simulink model "modeloKevin"  (R2017b)
settings: Solver=VariableStepAuto  StartTime=0.0  StopTime=200  RelTol=1e-3
values from neighbouring files (symbols this model uses):
  Awr = 0.0058    [variablesms.m]
  b = 0.0000000001    (= 1e-10)    [variablesms.m]
  Bi = 0.1    [variablesms.m]
  c = 0.012    [variablesms.m]
  CargaR = 1000    [variablesms.m]
  cpg = 1006    [variablesms.m]
  cpv = 1873.3    [variablesms.m]
  cpw = 4227    [variablesms.m]
  dg = 1.23    [variablesms.m]
  dv = 14.71    [variablesms.m]
  dw = 1000    [variablesms.m]
  F1 = 0.001    [variablesms.m]
  F2 = 0.001    [variablesms.m]
  fve = 60/(2*pi())    [variablesms.m]
  h = 1000    [variablesms.m]
  J = 0.004    [variablesms.m]
  Ji = 1.72    [variablesms.m]
  Kb = 6.2    [variablesms.m]
  Kp = 5.6627    [variablesms.m]
  l = 0.06    [variablesms.m]
  L_d = 38e-3    (= 0.038)    [variablesms.m]
  L_q = 9.03e-3    (= 0.00903)    [variablesms.m]
  Lambda = 0.48    [variablesms.m]
  P = 1    [variablesms.m]
  Patm = 101.325    [variablesms.m]
  r = 0.02    [variablesms.m]
  Rg = 0.287    [variablesms.m]
  Ri = 0.973    [variablesms.m]
  rp = 0.015    [variablesms.m]
  Rs = 1.649    [variablesms.m]
  Tcold = 300    [variablesms.m]
  Thot = 600    [variablesms.m]
  V1 = 0.001    [variablesms.m]
  V2 = 0.001    [variablesms.m]
undefined symbols (not defined in the file or in its folder): sigbuilder_block
libraries: powerlib_meascontrol x1, simulink x1
settings Model: Creator=Osorio  LastModifiedBy=Hp 14
settings CodeAppCC: StateflowObjectComments=on

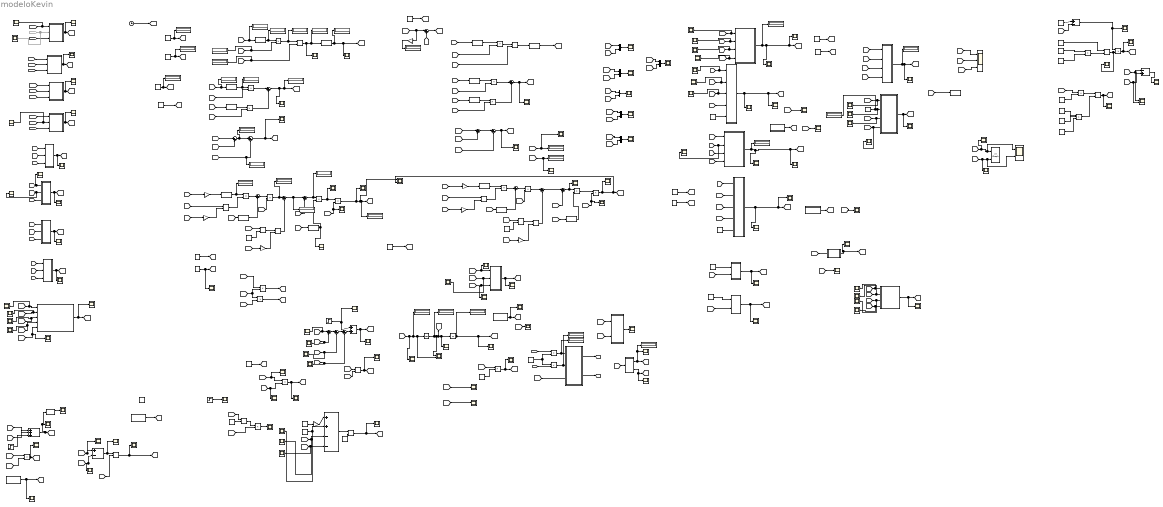
== system modeloKevin ==
  note: RORE AMARILLO
      | TORC AZUL
  note: ECUACION 30
  note: ECUACION 29
  note: ECUACION 27
  note: ECUACION 28
  note: ECUACION 24
  note: ECUACIO 25
  note: ECUACION 22
  note: ECUACION 23
  note: ecuacion 21
  note: ecuacion20
  note: ECUACIONES 15 16 17 18 19
  note: ECUACION 14
  note: ECUACION 13
  note: ECUACION12
  note: ECUACION 11
  note: ECUACION 10
  note: ECUACION 9
  note: ECUACION 8
  note: ECUACION6
  note: ECUACION 7
  note: MODELO TERMODINAMICO
  note: para expasion
  note: para compresion
  note: MODEO TERMICO
  note: MODELO DEL REGENERADOR
  note: MODELO MECANICO
  note: ECUACION 1
  note: MODELO DEL REGENERADOR
  note: ECUACION 2
  note: ECUACION 2
  note: ECUACION 2
  note: ECUACION 2
  note: ECUACION 31
  (-h)/(dg*cpg : Constant  Value=-h/(dg*cpg)
  (h*A)/(dg*cpg) : Constant  Value=(h*Awr)/(dg*cpg)
  Ap : Constant  Value=0.0007068
  Clock : Clock
  Constant : Constant  Value=r
  Constant1 : Constant  Value=l
  Constant{3,5..6,16} (4 alike) : Constant  Value=2
  Constant2 : Constant  Value=Patm
  Constant4 : Constant  Value=r
  Constant7 : Constant  Value=l
  Constant8 : Constant  Value=fve
  Constant9 : Constant  Value=CargaR
  Display{,1..32} (33 alike) : Display
  Divide{,1,3,5,8,10,15,17..18,21,24} (11 alike) : Product  Inputs=*/
  Divide{2,4,6..7,9,11..14,16,19..20,23,25..26} (15 alike) : Product  Inputs=**
  Divide22 : Product  Inputs=***
  Exp : Math  Operator=pow  SaturateOnIntegerOverflow=on
  F2/(V2*dv) : Constant  Value=F2/(V2*dv)
  Fcn : Fcn  Expr=sin(u)
  Fcn1 : Fcn  Expr=asin(u)
  Fcn10 : Fcn  Expr=tan(u)
  Fcn11 : Fcn  Expr=tan(u)
  Fcn{2..4,6..9,12..13} (9 alike) : Fcn  Expr=cos(u)
  Fcn5 : Fcn  Expr=asin(u)
  From111 : From  Commented=on  GotoTag=T22
  Gain : Gain  Gain=2
  Gain{1..2,4..6} (5 alike) : Gain  Gain=4
  Gain3 : Gain  Gain=2
  Gain7 : Gain  Gain=180/pi
  Integrator2 : Integrator
  Integrator3 : Integrator
  MATLAB Function1 : MATLAB Function  TreatAsAtomicUnit=on
  MATLAB Function2 : MATLAB Function  TreatAsAtomicUnit=on
  MATLAB Function3 : MATLAB Function  TreatAsAtomicUnit=on
  MATLAB Function4 : MATLAB Function  TreatAsAtomicUnit=on
  MATLAB Function5 : MATLAB Function  TreatAsAtomicUnit=on
  MATLAB Function6 : MATLAB Function  TreatAsAtomicUnit=on
  MATLAB Function7 : MATLAB Function  TreatAsAtomicUnit=on
  Math Function : Math  Operator=pow  SaturateOnIntegerOverflow=on
  Math Function1 : Math  Operator=pow  SaturateOnIntegerOverflow=on
  Mux{,1..5} (6 alike) : Mux  Inputs=2
  PLL : powerlib_meascontrol/PLL/PLL  Fmin=45  Par_Init=[0, 60]  ParK=[180, 3200, 1]  TcD=1e-4  MaxRateChangeFreq=12  FilterCutOffFreq=25  Ts=0  AGC=on
      settings: SourceProductName=Simscape Power Systems  SourceProductBaseCode=PS
  Product{,1..9} (10 alike) : Product
  Rg1 : Constant  Value=V1
  Rg3 : Constant  Value=V1
  Rg4 : Constant  Value=cpw
  Rg5 : Constant  Value=h
  Rg6 : Constant  Value=F1
  Rg7 : Constant  Value=V1
  Rg8 : Constant  Value=dw
  Scope{,1..30,32..42,44..57,59..73,75..76,78..125} (121 alike) : Scope
  Scope{31,58,74,77} (4 alike) : Scope  NumInputPorts=2
  Scope43 : Scope  NumInputPorts=3
  Signal Builder : Subsystem  Tag=STV Subsys  LoadFcn=sigbuilder_block('load');  StartFcn=sigbuilder_block('start');  StopFcn=sigbuilder_block('stop');  ClipboardFcn=sigbuilder_block('clipboard');  mask(Sigbuilder block){tuvar=[0:10]}
      mask help: Simulink:masks:SigbuilderBlock_MD
      mask init:
      | if ~strcmp(get_param(bdroot(gcbh),'SimulationStatus'),'stopped') tuvar = sigbuilder_block('maskInit'); end
      settings: CopyFcn=sigbuilder_block('copy');  DeleteFcn=sigbuilder_block('delete');  ModelCloseFcn=sigbuilder_block('modelClose');  PreSaveFcn=sigbuilder_block('preSave');  PauseFcn=sigbuilder_block('pause');  ContinueFcn=sigbuilder_block('continue');  NameChangeFcn=sigbuilder_block('namechange');  OpenFcn=sigbuilder_block('open',[169.5 67.5 550.5 359.25 ]);  CloseFcn=sigbuilder_block('close');
      mask Display: plot(0, 0, 100, 100,[2, 2, 32, 32, 2], [68, 8, 8, 68, 68],[32, 2], [38, 38], [32, 19, 2],[53, 60, 44], [32, 17, 17, 2],[16, 16, 31, 31]);txt = getActiveGroup(gcbh);text(2, 100, txt,'verticalAlignment', 'top');
  Signal Builder1 : Subsystem  Tag=STV Subsys  LoadFcn=sigbuilder_block('load');  StartFcn=sigbuilder_block('start');  StopFcn=sigbuilder_block('stop');  ClipboardFcn=sigbuilder_block('clipboard');  mask(Sigbuilder block){tuvar=[0:10]}
      mask help: Simulink:masks:SigbuilderBlock_MD
      mask init:
      | if ~strcmp(get_param(bdroot(gcbh),'SimulationStatus'),'stopped') tuvar = sigbuilder_block('maskInit'); end
      settings: CopyFcn=sigbuilder_block('copy');  DeleteFcn=sigbuilder_block('delete');  ModelCloseFcn=sigbuilder_block('modelClose');  PreSaveFcn=sigbuilder_block('preSave');  PauseFcn=sigbuilder_block('pause');  ContinueFcn=sigbuilder_block('continue');  NameChangeFcn=sigbuilder_block('namechange');  OpenFcn=sigbuilder_block('open',[169.5 67.5 550.5 359.25 ]);  CloseFcn=sigbuilder_block('close');
      mask Display: plot(0, 0, 100, 100,[2, 2, 32, 32, 2], [68, 8, 8, 68, 68],[32, 2], [38, 38], [32, 19, 2],[53, 60, 44], [32, 17, 17, 2],[16, 16, 31, 31]);txt = getActiveGroup(gcbh);text(2, 100, txt,'verticalAlignment', 'top');
  Signal Builder2 : Subsystem  Tag=STV Subsys  LoadFcn=sigbuilder_block('load');  StartFcn=sigbuilder_block('start');  StopFcn=sigbuilder_block('stop');  ClipboardFcn=sigbuilder_block('clipboard');  mask(Sigbuilder block){tuvar=[0:10]}
      mask help: Simulink:masks:SigbuilderBlock_MD
      mask init:
      | if ~strcmp(get_param(bdroot(gcbh),'SimulationStatus'),'stopped') tuvar = sigbuilder_block('maskInit'); end
      settings: CopyFcn=sigbuilder_block('copy');  DeleteFcn=sigbuilder_block('delete');  ModelCloseFcn=sigbuilder_block('modelClose');  PreSaveFcn=sigbuilder_block('preSave');  PauseFcn=sigbuilder_block('pause');  ContinueFcn=sigbuilder_block('continue');  NameChangeFcn=sigbuilder_block('namechange');  OpenFcn=sigbuilder_block('open',[169.5 67.5 550.5 359.25 ]);  CloseFcn=sigbuilder_block('close');
      mask Display: plot(0, 0, 100, 100,[2, 2, 32, 32, 2], [68, 8, 8, 68, 68],[32, 2], [38, 38], [32, 19, 2],[53, 60, 44], [32, 17, 17, 2],[16, 16, 31, 31]);txt = getActiveGroup(gcbh);text(2, 100, txt,'verticalAlignment', 'top');
  Signal Builder3 : Subsystem  Tag=STV Subsys  LoadFcn=sigbuilder_block('load');  StartFcn=sigbuilder_block('start');  StopFcn=sigbuilder_block('stop');  ClipboardFcn=sigbuilder_block('clipboard');  mask(Sigbuilder block){tuvar=[0:10]}
      mask help: Simulink:masks:SigbuilderBlock_MD
      mask init:
      | if ~strcmp(get_param(bdroot(gcbh),'SimulationStatus'),'stopped') tuvar = sigbuilder_block('maskInit'); end
      settings: CopyFcn=sigbuilder_block('copy');  DeleteFcn=sigbuilder_block('delete');  ModelCloseFcn=sigbuilder_block('modelClose');  PreSaveFcn=sigbuilder_block('preSave');  PauseFcn=sigbuilder_block('pause');  ContinueFcn=sigbuilder_block('continue');  NameChangeFcn=sigbuilder_block('namechange');  OpenFcn=sigbuilder_block('open',[6 6 1012.5 506.25 ]);  CloseFcn=sigbuilder_block('close');
      mask Display: plot(0, 0, 100, 100,[2, 2, 32, 32, 2], [68, 8, 8, 68, 68],[32, 2], [38, 38], [32, 19, 2],[53, 60, 44], [32, 17, 17, 2],[16, 16, 31, 31]);txt = getActiveGroup(gcbh);text(2, 100, txt,'verticalAlignment', 'top');
  Signal Builder4 : Subsystem  Tag=STV Subsys  LoadFcn=sigbuilder_block('load');  StartFcn=sigbuilder_block('start');  StopFcn=sigbuilder_block('stop');  ClipboardFcn=sigbuilder_block('clipboard');  mask(Sigbuilder block){tuvar=[0:10]}
      mask help: Simulink:masks:SigbuilderBlock_MD
      mask init:
      | if ~strcmp(get_param(bdroot(gcbh),'SimulationStatus'),'stopped') tuvar = sigbuilder_block('maskInit'); end
      settings: CopyFcn=sigbuilder_block('copy');  DeleteFcn=sigbuilder_block('delete');  ModelCloseFcn=sigbuilder_block('modelClose');  PreSaveFcn=sigbuilder_block('preSave');  PauseFcn=sigbuilder_block('pause');  ContinueFcn=sigbuilder_block('continue');  NameChangeFcn=sigbuilder_block('namechange');  OpenFcn=sigbuilder_block('open',[6 30 1428 681.75 ]);  CloseFcn=sigbuilder_block('close');
      mask Display: plot(0, 0, 100, 100,[2, 2, 32, 32, 2], [68, 8, 8, 68, 68],[32, 2], [38, 38], [32, 19, 2],[53, 60, 44], [32, 17, 17, 2],[16, 16, 31, 31]);txt = getActiveGroup(gcbh);text(2, 100, txt,'verticalAlignment', 'top');
  Step : Step  Time=70  Before=0.0001  After=0.00015  SampleTime=1
  Step1 : Step  Time=2  Before=0.7  After=0  SampleTime=1
  Step3 : Step  Time=2  Before=0.7  After=0  SampleTime=1
  Subsystem1 : Subsystem
  Subsystem10 : Subsystem
  Subsystem11 : Subsystem
  Subsystem12 : Subsystem
  Subsystem13 : Subsystem
  Subsystem14 : Subsystem
  Subsystem15 : Subsystem
  Subsystem16 : Subsystem
  Subsystem2 : Subsystem
  Subsystem3 : Subsystem
  Subsystem4 : Subsystem
  Subsystem5 : Subsystem
  Subsystem6 : Subsystem
  Subsystem7 : Subsystem
  Subsystem8 : Subsystem
  Subsystem9 : Subsystem
  Sum{,3,5..7,9,12,17..19} (10 alike) : Sum  Inputs=|++
  Sum1 : Sum  Inputs=|++--
  Sum{2,8,10..11,13..14,16,21} (8 alike) : Sum  Inputs=|+-
  Sum15 : Sum  Inputs=|-+
  Sum20 : Sum  Inputs=|+++
  Sum4 : Sum  Inputs=|-+
  Tcold2 : Constant  Value=Tcold
  Thot : Constant  Value=Thot
  Thot1 : Constant  Value=Tcold
  To Workspace : ToWorkspace  VariableName=simout  SaveFormat=Timeseries  SampleTime=-1
  XY Graph : simulink/Sinks/XY Graph  xmin=0.00003  xmax=0.00009  ymin=0  ymax=900  st=-1
  Xreg : Constant  Value=0.04
  desfazamiento : Constant  Value=1.57079
  desfazamiento1 : Constant  Value=b
  desfazamiento3 : Constant  Value=c
  desfazamiento4 : Constant  Value=J
  h/V2*dv*cpv) : Constant  Value=h/(V2*dv*cpv)
  h/V2*dv*cpv)1 : Constant  Value=rp
  h/V2*dv*cpv)2 : Constant  Value=rp
  mg : Constant  Value=0.0002
  mg1 : Constant  Value=Rg
  tag scope: Id=global, Iq=global
  wires:
  (h*A)/(dg*cpg)/1 -> [C1]
  (-h)/(dg*cpg/1 -> Display1/1, [c2]
  [Acilc] -> Scope44/1, Subsystem2/1(In1)
  [c2] -> Scope45/1, Subsystem2/2(In2)
  [Vg] -> Scope46/1, Subsystem2/3(In3)
  [T11] -> Scope47/1, Subsystem2/4(In4)
  F2/(V2*dv)/1 -> [c5]
  h/V2*dv*cpv)/1 -> [c6]
  Xreg/1 -> [Xreg]
  Ap/1 -> [Ap]
  [Xc] -> Subsystem7/1(In1)
  [Xe] -> Subsystem7/2(In2)
  [Xreg] -> Subsystem7/3(In3)
  [Ap] -> Subsystem7/4(In4)
  Subsystem7/1(Out1) -> Display10/1, Scope40/1, [Vg]
  [Tge] -> Subsystem5/1(In1)
  [Acile] -> Subsystem5/2(In2)
  [c6] -> Subsystem5/3(In3)
  [c5] -> Subsystem5/4(In4)
  Thot/1 -> Subsystem5/5(In5)
  h/V2*dv*cpv)1/1 -> Subsystem6/1(In1)
  [Xe] -> Subsystem6/2(In2)
  Subsystem6/1(Out1) -> Scope41/1, [Acile]
  h/V2*dv*cpv)2/1 -> Subsystem8/1(In1)
  [Xc] -> Subsystem8/2(In2)
  Subsystem8/1(Out1) -> Scope42/1, [Acilc]
  [mg] -> Scope79/1, Subsystem9/1(In1)
  mg1/1 -> Display19/1, Scope78/1, Subsystem9/2(In2)
  [TG] -> Scope66/1, Subsystem9/3(In3)
  [Vg] -> Scope65/1, Subsystem9/4(In4)
  Subsystem9/1(Out1) -> Scope64/1, [Pg]
  Sum7/1 -> Divide4/1
  [k] -> Fcn13/1
  Mux/1 -> Scope7/1
  [l] -> Product5/2
  [r] -> Display12/1, Product/2
  [b] -> Divide12/2
  Sum16/1 -> Sum17/1
  [torc] -> Mux3/2
  Fcn8/1 -> Display17/1, Product6/1
  Product3/1 -> Divide1/1
  Divide3/1 -> Product6/2
  Divide6/1 -> Scope61/1, Divide2/1
  Mux3/1 -> Scope18/1
  [tore] -> Mux3/1
  Fcn6/1 -> Product4/1
  [cc] -> Mux5/2
  Constant6/1 -> Math Function1/2
  Mux4/1 -> Scope19/1
  [Xe] -> Scope10/1, Display27/1
  [r] -> Divide4/2
  [r] -> Divide3/1
  Gain2/1 -> Divide5/2
  Fcn3/1 -> Product2/1
  Divide5/1 -> Sum8/2
  [Fg] -> Scope33/1, Divide2/2
  Sum10/1 -> Scope4/1, [Xe]
  [FIe] -> Mux4/1
  Sum8/1 -> Display21/1, Sum9/1
  [FIc] -> Mux2/1
  Gain/1 -> Fcn8/1
  Mux2/1 -> Scope11/1
  Fcn12/1 -> Product7/1
  [Xc] -> Mux1/2
  Constant1/1 -> Display8/1, [l]
  Gain7/1 -> Display5/1
  [FIc] -> Fcn7/1
  Divide12/1 -> [torf]
  [theta] -> Mux2/2
  Constant/1 -> Display/1, [r]
  [theta] -> Sum4/2
  [l] -> Sum18/2
  Product4/1 -> Sum5/1
  [FIe] -> Mux/1
  [r] -> Sum18/1
  Divide13/1 -> [torq]
  Sum18/1 -> Display31/1, Sum10/1
  Fcn9/1 -> Sum7/2
  Product2/1 -> Sum3/2
  Divide11/1 -> Divide7/1
  [l] -> Product2/2
  Divide10/1 -> Sum16/2
  [r] -> Product1/2
  Divide/1 -> Scope2/1, Display23/1, Fcn1/1
  [theta] -> Display11/1, Fcn/1
  Fcn/1 -> Display24/1, Product/1
  Math Function1/1 -> Divide10/1
  [cc] -> Sum11/2
  Math Function/1 -> Divide5/1
  Fcn2/1 -> Display15/1, Product1/1
  [l] -> Gain1/1
  [r] -> Divide8/1
  Fcn7/1 -> Product5/1
  Sum9/1 -> Display22/1, Divide6/1
  Mux5/1 -> Scope20/1
  [c] -> Divide13/1
  Product5/1 -> Sum5/2
  [Fg] -> Scope35/1, Divide7/2
  Fcn1/1 -> Display7/1, Scope21/1, [FIe]
  [FIc] -> Mux4/2
  Gain4/1 -> Divide8/2
  [theta] -> Mux/2
  Fcn4/1 -> Product3/1
  [r] -> Divide9/2
  [ce] -> Display25/1, Sum10/2
  Gain3/1 -> Fcn12/1
  [r] -> Sum12/1
  Divide1/1 -> Fcn5/1
  [l] -> Sum9/2
  [theta] -> Fcn9/1
  [fi] -> Gain7/1, Sum4/1
  [l] -> Sum12/2
  [ce] -> Mux5/1
  [r] -> Product4/2
  [FIe] -> Fcn10/1
  Sum4/1 -> [k]
  [l] -> Gain5/1
  Divide4/1 -> Display20/1, Sum8/1
  Divide2/1 -> Scope5/1, Scope74/1, Display18/1, [tore]
  Fcn13/1 -> Sum6/2
  [l] -> Gain4/1
  [l] -> Display13/1, Divide/2
  Fcn5/1 -> [FIc]
  [w] -> Divide13/2, Divide12/1
  [theta] -> Gain/1
  [l] -> Sum17/2
  [FIe] -> Fcn11/1
  [r] -> Product3/2
  [FIe] -> Fcn3/1
  Mux1/1 -> Scope17/1
  Sum3/1 -> Scope3/1, Display16/1, [ce]
  Product/1 -> Display26/1, Divide/1
  [theta] -> Display14/1, Fcn2/1
  [Xe] -> Mux1/1
  [l] -> Divide1/2
  Sum11/1 -> Scope28/1, [Xc]
  Fcn11/1 -> Divide11/2
  Divide8/1 -> Product7/2
  desfazamiento3/1 -> Scope116/1, [c]
  [k] -> Gain3/1
  Gain5/1 -> Divide10/2
  Sum5/1 -> Scope27/1, [cc]
  [k] -> Fcn6/1
  Divide7/1 -> Scope74/2, [torc], Scope36/1
  [k] -> Fcn4/1
  Product7/1 -> Sum6/1
  Sum6/1 -> Divide9/1
  desfazamiento/1 -> [fi]
  Sum17/1 -> Scope60/1, Divide11/1
  [l] -> Gain2/1
  Gain1/1 -> Divide3/2
  Sum12/1 -> Sum11/1
  Fcn10/1 -> Scope1/1, Divide6/2
  Product6/1 -> Sum7/1
  [r] -> Math Function1/1
  Constant5/1 -> Math Function/2
  [r] -> Math Function/1
  desfazamiento1/1 -> [b]
  [Xc] -> Scope105/1, Display28/1
  Divide9/1 -> Sum16/1
  Product1/1 -> Sum3/1
  Constant2/1 -> [Patm]
  [w] -> Scope115/1, Divide16/1
  [c] -> Scope114/1, Divide16/2
  Divide16/1 -> Scope73/1, [Pn]
  [Xc] -> Scope51/1, Sum1/4
  Gain6/1 -> Sum1/1
  Constant16/1 -> Divide15/2
  Divide15/1 -> Scope48/1, [Xg]
  Sum1/1 -> Divide15/1
  Constant4/1 -> Gain6/1
  [Xe] -> Scope50/1, Sum1/3
  Constant7/1 -> Scope49/1, Sum1/2
  [Pn] -> Scope22/1
  [Xg] -> Scope23/1
  Sum14/1 -> Sum19/2
  Sum19/1 -> Scope32/1, [TORT]
  [torc] -> Sum/2, Scope13/1
  [J] -> Divide18/2
  [tore] -> Sum/1, Scope12/1
  Divide18/1 -> Scope34/1, [ACE]
  Sum13/1 -> Sum14/1
  [torq] -> Sum13/2, Scope14/1
  [TORT] -> Divide18/1
  Sum/1 -> Sum13/1
  [torf] -> Sum14/2, Scope15/1
  Integrator3/1 -> Scope9/1, [theta], Display9/1
  Integrator2/1 -> Display30/1, Scope31/1, [w], Scope6/1, Integrator3/1
  [ACE2] -> Scope8/1, Display29/1, Scope31/2, Integrator2/1
  desfazamiento4/1 -> [J]
  MATLAB Function3/1(y) -> Scope24/1, [pcs]
  [pcs] -> Scope/1
  [Pg] -> Scope63/1, Subsystem12/1(In1)
  [Patm] -> Scope96/1, Subsystem12/2(In2)
  [Ap] -> Scope62/1, Subsystem12/3(In3)
  Subsystem12/1(Out1) -> Scope52/1, [Fg]
  Step3/1 -> Scope30/1, Sum19/1
  Clock/1 -> [t]
  [theta] -> MATLAB Function3/1(tetha)
  Signal Builder/1(Signal 1) -> Scope37/1, [thetaa]
  [thetaa] -> Scope25/1
  [pcs] -> Scope72/1, MATLAB Function5/4(pcs)
  [Tgw] -> Scope70/1, MATLAB Function5/3(Tgw)
  [T22] -> Scope69/1, MATLAB Function5/2(T22)
  [T11] -> Scope68/1, MATLAB Function5/1(T11)
  [Vg] -> Scope43/1
  [Acile] -> Scope43/2
  [Acilc] -> Scope43/3
  Rg7/1 -> Divide14/1
  Rg8/1 -> Divide14/2
  Divide14/1 -> Divide17/2
  Rg6/1 -> Divide17/1
  Tcold2/1 -> Sum2/1
  [Tgc] -> Sum2/2
  Divide17/1 -> Scope56/1, Divide19/2
  Sum2/1 -> Scope57/1, Divide19/1
  Divide19/1 -> Scope54/1, [P1]
  [Acilc] -> Divide20/1
  Rg5/1 -> Divide20/2
  Divide20/1 -> Divide21/1
  Rg4/1 -> Divide22/1
  Rg1/1 -> Divide22/2
  Rg3/1 -> Divide22/3
  Divide22/1 -> Divide21/2
  Divide21/1 -> Scope55/1, [P2]
  [P1] -> Scope58/1, Sum15/1
  [P2] -> Scope58/2, Sum15/2
  Sum15/1 -> Scope53/1
  MATLAB Function5/1(Y) -> Scope39/1, [TG]
  [T11] -> Scope59/1
  Signal Builder1/1(Signal 2) -> [T2]
  Signal Builder2/1(Signal 2) -> [T1]
  [T22] -> Subsystem10/4(In4)
  [c2] -> Scope80/1, Subsystem10/2(In2)
  [Vg] -> Subsystem10/3(In3)
  [Acile] -> Subsystem10/1(In1)
  [Vg] -> To Workspace/1
  [Vg] -> Scope75/1, Scope77/1, XY Graph/1
  [Pg] -> Scope76/1, Scope77/2, XY Graph/2
  Thot1/1 -> Subsystem4/5(In5)
  [c5] -> Subsystem4/4(In4)
  [c6] -> Scope108/1, Subsystem4/3(In3)
  [Acilc] -> Scope107/1, Subsystem4/2(In2)
  [Tgc] -> Scope106/1, Subsystem4/1(In1)
  [T11] -> Scope88/1, MATLAB Function1/1(T1)
  [T11] -> MATLAB Function7/1(T1)
  [t] -> MATLAB Function7/3(t)
  [t] -> MATLAB Function4/3(t)
  [t] -> MATLAB Function1/3(t)
  From111/1 -> Scope89/1, MATLAB Function1/2(T2)
  [T22] -> MATLAB Function4/2(T2)
  [T22] -> Scope109/1, MATLAB Function7/2(T2)
  MATLAB Function7/1(y4) -> Scope85/1, [TW4]
  [t] -> MATLAB Function2/3(t)
  [T11] -> MATLAB Function4/1(T1)
  [T11] -> MATLAB Function2/1(T1)
  [T22] -> MATLAB Function2/2(T2)
  MATLAB Function2/1(y2) -> Scope16/1, [TW2]
  MATLAB Function1/1(y1) -> Scope26/1, [TW1]
  MATLAB Function4/1(y3) -> Scope82/1, [TW3]
  [Xg] -> Scope90/1, MATLAB Function6/5(Xg)
  [Tg4] -> Scope94/1, MATLAB Function6/4(T4)
  [C1] -> Subsystem13/3(In3)
  [Tg3] -> Scope93/1, MATLAB Function6/3(T3)
  [C1] -> Subsystem1/3(In3)
  [Vg] -> Subsystem1/2(In2)
  Subsystem1/1(Out1) -> Scope67/1, [Tg1]
  [TW1] -> Subsystem1/1(In1)
  [TW4] -> Subsystem13/1(In1)
  [Vg] -> Subsystem13/2(In2)
  [TW3] -> Subsystem11/1(In1)
  [Tg1] -> Scope91/1, MATLAB Function6/1(T1)
  [Tg2] -> Scope92/1, MATLAB Function6/2(T2)
  MATLAB Function6/1(Twg) -> Scope87/1, [Tgw]
  Subsystem13/1(Out1) -> Scope86/1, [Tg4]
  Subsystem3/1(Out1) -> Scope83/1, [Tg2]
  [Vg] -> Subsystem11/2(In2)
  [Vg] -> Scope104/1, Subsystem3/2(In2)
  [C1] -> Subsystem11/3(In3)
  Subsystem11/1(Out1) -> Scope84/1, [Tg3]
  [C1] -> Subsystem3/3(In3)
  [TW2] -> Scope103/1, Subsystem3/1(In1)
  Subsystem2/1(Out1) -> Scope98/1, [Tgc], Scope99/1, Display2/1
  [T1] -> Scope38/1
  [T2] -> Scope97/1
  Subsystem4/1(Out1) -> Scope100/1, [T11], Scope81/1
  Subsystem10/1(Out1) -> Display4/1, Scope101/1, [Tge], Scope71/1
  Subsystem5/1(Out1) -> Scope102/1, [T22], Scope29/1
  Step/1 -> Scope95/1
  [tore] -> Sum20/1
  [torc] -> Sum20/2
  Sum20/1 -> PLL/1, Scope112/1, [tortepositivo]
  [tortepositivo] -> Divide23/1
  [factort] -> Divide23/2
  Divide23/1 -> Scope113/1, [torquenegativo]
  [tortepositivo] -> Scope119/1, Sum21/1
  [torquenegativo] -> Scope118/1, Sum21/2
  Sum21/1 -> Scope120/1, Divide24/1
  [J] -> Divide24/2
  Signal Builder3/1(Signal 2) -> Scope110/1, [factort]
  Divide24/1 -> Scope111/1, [ACE2]
  Step1/1 -> Sum20/3
  Constant3/1 -> Exp/2
  [w] -> Exp/1
  Exp/1 -> Divide25/1
  [c] -> Divide25/2
  Divide25/1 -> Scope117/1
  [w] -> Divide26/1
  Constant8/1 -> Divide26/2
  Divide26/1 -> Scope121/1, [rpm]
  Signal Builder4/1(Signal 2) -> [mg]
  [Id] -> Product9/1
  Product9/1 -> Display3/1, Subsystem14/1(Vd)
  [Iq] -> Product8/2
  Product8/1 -> Display6/1, Subsystem14/2(Vq)
  Constant9/1 -> Product8/1, Product9/2
  Subsystem14/2(Iq) -> [Iq]
  Subsystem14/1(Id) -> [Id]
  [w] -> Subsystem14/3(We)
  [Iq] -> Subsystem15/1(Iq)
  [Id] -> Subsystem15/2(Id)
  Subsystem15/1(Te) -> Scope122/1
  Subsystem16/1(Out1) -> Display32/1, Scope123/1, [Pout]
  Subsystem16/2(Out2) -> [TEout], Scope124/1
  [w] -> Subsystem16/1(In1)
  PLL/1 -> Scope125/1

== system modeloKevin/Signal Builder ==
  Demux : Demux  Tag=STV Demux  Outputs=1
  FromWs : FromWorkspace  Tag=STV FromWs  VariableName=tuvar  SampleTime=0
      SigBuilderData=|
      | common.afterFinalStr = 'Extrapolate'
      | common.sampleTime = 0
      | dataSet.timeRange = [0 10]
      | dataSet.name = 'Group 1'
      | sbobj.Groups.Name = 'Group 1'
      | sbobj.Groups.Signals.Name = 'Signal 1'
      | sbobj.Groups.Signals.XData = [0 10]
      | sbobj.Groups.Signals.YData = [0.1 50]
  Signal 1 : Outport  Tag=STV Outport
  wires:
  FromWs/1 -> Demux/1
  Demux/1 -> Signal 1/1

== system modeloKevin/Signal Builder1 ==
  Demux : Demux  Tag=STV Demux  Outputs=1
  FromWs : FromWorkspace  Tag=STV FromWs  VariableName=tuvar  SampleTime=0
      SigBuilderData=|
      | common.afterFinalStr = 'Extrapolate'
      | common.sampleTime = 0
      | dataSet.timeRange = [0 10]
      | dataSet.name = 'Group 1'
      | sbobj.Groups.Name = 'Group 1'
      | sbobj.Groups.Signals.Name = 'Signal 2'
      | sbobj.Groups.Signals.XData = [0 5 10]
      | sbobj.Groups.Signals.YData = [300 311.5 320]
  Signal 2 : Outport  Tag=STV Outport
  wires:
  FromWs/1 -> Demux/1
  Demux/1 -> Signal 2/1

== system modeloKevin/Signal Builder2 ==
  Demux : Demux  Tag=STV Demux  Outputs=1
  FromWs : FromWorkspace  Tag=STV FromWs  VariableName=tuvar  SampleTime=0
      SigBuilderData=|
      | common.afterFinalStr = 'Extrapolate'
      | common.sampleTime = 0
      | dataSet.timeRange = [0 10]
      | dataSet.name = 'Group 1'
      | sbobj.Groups.Name = 'Group 1'
      | sbobj.Groups.Signals.Name = 'Signal 2'
      | sbobj.Groups.Signals.XData = [0 5 10]
      | sbobj.Groups.Signals.YData = [300 400 400]
  Signal 2 : Outport  Tag=STV Outport
  wires:
  FromWs/1 -> Demux/1
  Demux/1 -> Signal 2/1

== system modeloKevin/Signal Builder3 ==
  Demux : Demux  Tag=STV Demux  Outputs=1
  FromWs : FromWorkspace  Tag=STV FromWs  VariableName=tuvar  SampleTime=0
      SigBuilderData=|
      | common.afterFinalStr = 'Extrapolate'
      | common.sampleTime = 0
      | dataSet.timeRange = [0 500]
      | dataSet.name = 'Group 1'
      | sbobj.Groups.Name = 'Group 1'
      | sbobj.Groups.Signals.Name = 'Signal 2'
      | sbobj.Groups.Signals.XData = [0 8 9 500]
      | sbobj.Groups.Signals.YData = [0 0 1.002 1]
      | sbobj.Groups.TimeRange = [0 500]
  Signal 2 : Outport  Tag=STV Outport
  wires:
  FromWs/1 -> Demux/1
  Demux/1 -> Signal 2/1

== system modeloKevin/Signal Builder4 ==
  Demux : Demux  Tag=STV Demux  Outputs=1
  FromWs : FromWorkspace  Tag=STV FromWs  VariableName=tuvar  SampleTime=0
      SigBuilderData=|
      | common.afterFinalStr = 'Extrapolate'
      | common.sampleTime = 0
      | dataSet.timeRange = [0 500]
      | dataSet.name = 'Group 1'
      | sbobj.Groups.Name = 'Group 1'
      | sbobj.Groups.Signals.Name = 'Signal 2'
      | sbobj.Groups.Signals.XData = [0 50 51 500]
      | sbobj.Groups.Signals.YData = [0.0002 0.0002 0.0003 0.0003]
      | sbobj.Groups.TimeRange = [0 500]
  Signal 2 : Outport  Tag=STV Outport
  wires:
  FromWs/1 -> Demux/1
  Demux/1 -> Signal 2/1

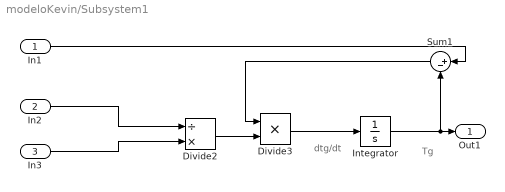
== system modeloKevin/Subsystem1 ==
  note: Tg
  note: dtg/dt
  In1 : Inport
  In2 : Inport  Port=2
  In3 : Inport  Port=3
  Divide2 : Product  Inputs=/*
  Divide3 : Product  Inputs=**
  Integrator : Integrator
  Sum1 : Sum  Inputs=|+-
  Out1 : Outport
  wires:
  Sum1/1 -> Divide3/1
  Integrator/1 -> Sum1/2, Out1/1
  In1/1 -> Sum1/1
  Divide2/1 -> Divide3/2
  In3/1 -> Divide2/2
  In2/1 -> Divide2/1
  Divide3/1 -> Integrator/1

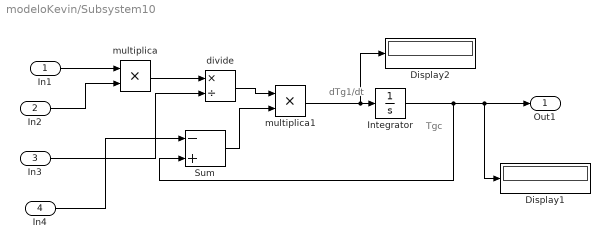
== system modeloKevin/Subsystem10 ==
  note: Tgc
  note: dTg1/dt
  In1 : Inport
  In2 : Inport  Port=2
  In3 : Inport  Port=3
  In4 : Inport  Port=4
  Display1 : Display
  Display2 : Display
  Integrator : Integrator
  Sum : Sum  Inputs=|-+
  divide : Product  Inputs=*/
  multiplica : Product  Inputs=**
  multiplica1 : Product  Inputs=**
  Out1 : Outport
  wires:
  In3/1 -> divide/2
  In1/1 -> multiplica/1
  multiplica1/1 -> Display2/1, Integrator/1
  In4/1 -> Sum/1
  Sum/1 -> multiplica1/2
  divide/1 -> multiplica1/1
  In2/1 -> multiplica/2
  multiplica/1 -> divide/1
  Integrator/1 -> Display1/1, Out1/1, Sum/2

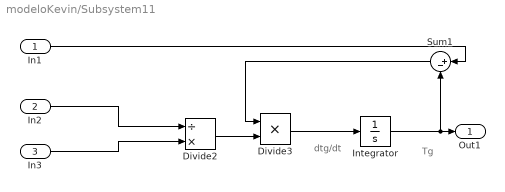
== system modeloKevin/Subsystem11 ==
  note: Tg
  note: dtg/dt
  In1 : Inport
  In2 : Inport  Port=2
  In3 : Inport  Port=3
  Divide2 : Product  Inputs=/*
  Divide3 : Product  Inputs=**
  Integrator : Integrator
  Sum1 : Sum  Inputs=|+-
  Out1 : Outport
  wires:
  Sum1/1 -> Divide3/1
  Integrator/1 -> Sum1/2, Out1/1
  In1/1 -> Sum1/1
  Divide2/1 -> Divide3/2
  In3/1 -> Divide2/2
  In2/1 -> Divide2/1
  Divide3/1 -> Integrator/1

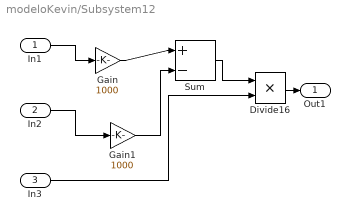
== system modeloKevin/Subsystem12 ==
  In1 : Inport
  In2 : Inport  Port=2
  In3 : Inport  Port=3
  Divide16 : Product  Inputs=**
  Gain : Gain  Gain=1000
  Gain1 : Gain  Gain=1000
  Sum : Sum  Inputs=|+-
  Out1 : Outport
  wires:
  In3/1 -> Divide16/2
  Divide16/1 -> Out1/1
  Sum/1 -> Divide16/1
  In1/1 -> Gain/1
  In2/1 -> Gain1/1
  Gain/1 -> Sum/1
  Gain1/1 -> Sum/2

== system modeloKevin/Subsystem13 ==
  note: Tg
  note: dtg/dt
  In1 : Inport
  In2 : Inport  Port=2
  In3 : Inport  Port=3
  Divide2 : Product  Inputs=/*
  Divide3 : Product  Inputs=**
  Integrator : Integrator
  Sum1 : Sum  Inputs=|+-
  Out1 : Outport
  wires:
  Sum1/1 -> Divide3/1
  Integrator/1 -> Sum1/2, Out1/1
  In1/1 -> Sum1/1
  Divide2/1 -> Divide3/2
  In3/1 -> Divide2/2
  In2/1 -> Divide2/1
  Divide3/1 -> Integrator/1

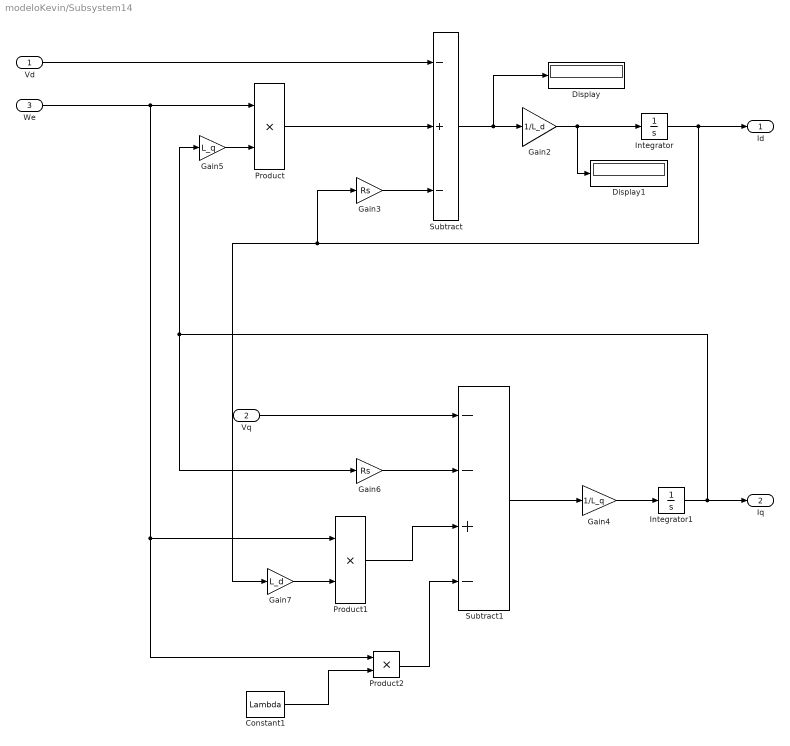
== system modeloKevin/Subsystem14 ==
  Vd : Inport
  Vq : Inport  Port=2
  We : Inport  Port=3
  Constant1 : Constant  Value=Lambda
  Display : Display
  Display1 : Display
  Gain2 : Gain  Gain=1/L_d
  Gain3 : Gain  Gain=Rs
  Gain4 : Gain  Gain=1/L_q
  Gain5 : Gain  Gain=L_q
  Gain6 : Gain  Gain=Rs
  Gain7 : Gain  Gain=L_d
  Integrator : Integrator
  Integrator1 : Integrator
  Product : Product
  Product1 : Product
  Product2 : Product
  Subtract : Sum  Inputs=-+-
  Subtract1 : Sum  Inputs=--+-
  Id : Outport
  Iq : Outport  Port=2
  wires:
  Integrator1/1 -> Gain6/1, Gain5/1, Iq/1
  We/1 -> Product/1, Product2/1, Product1/1
  Product1/1 -> Subtract1/3
  Gain7/1 -> Product1/2
  Product/1 -> Subtract/2
  Integrator/1 -> Id/1, Gain7/1, Gain3/1
  Gain4/1 -> Integrator1/1
  Gain2/1 -> Display1/1, Integrator/1
  Gain5/1 -> Product/2
  Subtract/1 -> Display/1, Gain2/1
  Subtract1/1 -> Gain4/1
  Vq/1 -> Subtract1/1
  Gain6/1 -> Subtract1/2
  Vd/1 -> Subtract/1
  Constant1/1 -> Product2/2
  Product2/1 -> Subtract1/4
  Gain3/1 -> Subtract/3

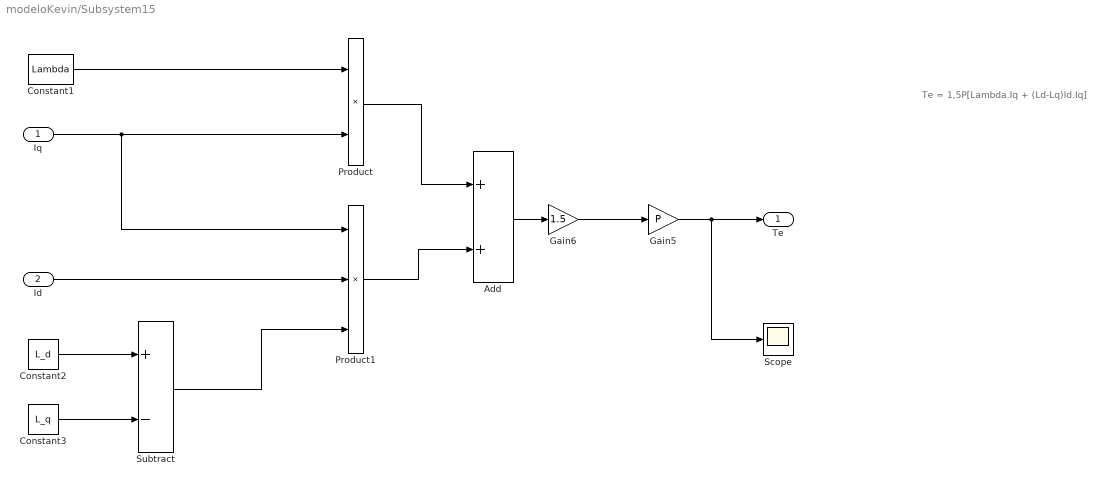
== system modeloKevin/Subsystem15 ==
  note: Te = 1,5P[Lambda.Iq + (Ld-Lq)Id.Iq]
  Iq : Inport
  Id : Inport  Port=2
  Add : Sum
  Constant1 : Constant  Value=Lambda
  Constant2 : Constant  Value=L_d
  Constant3 : Constant  Value=L_q
  Gain5 : Gain  Gain=P
  Gain6 : Gain  Gain=1.5
  Product : Product
  Product1 : Product  Inputs=3
  Scope : Scope
  Subtract : Sum  Inputs=+-
  Te : Outport
  wires:
  Product1/1 -> Add/2
  Iq/1 -> Product1/1, Product/2
  Constant1/1 -> Product/1
  Gain5/1 -> Scope/1, Te/1
  Subtract/1 -> Product1/3
  Id/1 -> Product1/2
  Gain6/1 -> Gain5/1
  Add/1 -> Gain6/1
  Product/1 -> Add/1
  Constant2/1 -> Subtract/1
  Constant3/1 -> Subtract/2

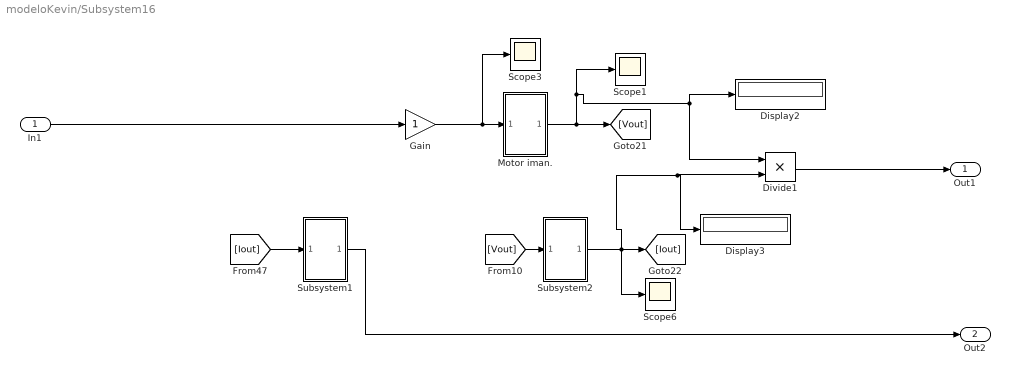
== system modeloKevin/Subsystem16 ==
  In1 : Inport
  Display2 : Display
  Display3 : Display
  Divide1 : Product  Inputs=**
  Gain : Gain
  Motor iman. : Subsystem
  Scope1 : Scope
  Scope3 : Scope
  Scope6 : Scope
  Subsystem1 : Subsystem
  Subsystem2 : Subsystem
  Out1 : Outport
  Out2 : Outport  Port=2
  wires:
  Motor iman./1(Out1) -> Divide1/1, Display2/1, Scope1/1, [Vout]
  Subsystem1/1(Out1) -> Out2/1
  [Iout] -> Subsystem1/1(In1)
  Subsystem2/1(Out1) -> Divide1/2, Display3/1, Scope6/1, [Iout]
  Divide1/1 -> Out1/1
  Gain/1 -> Scope3/1, Motor iman./1(In1)
  In1/1 -> Gain/1
  [Vout] -> Subsystem2/1(In1)

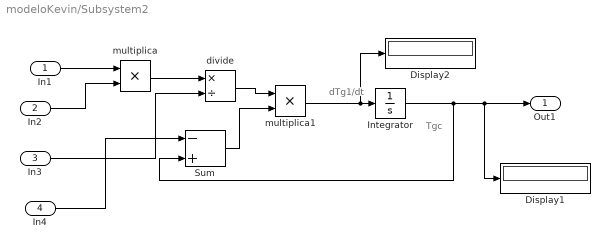
== system modeloKevin/Subsystem2 ==
  note: Tgc
  note: dTg1/dt
  In1 : Inport
  In2 : Inport  Port=2
  In3 : Inport  Port=3
  In4 : Inport  Port=4
  Display1 : Display
  Display2 : Display
  Integrator : Integrator
  Sum : Sum  Inputs=|-+
  divide : Product  Inputs=*/
  multiplica : Product  Inputs=**
  multiplica1 : Product  Inputs=**
  Out1 : Outport
  wires:
  In3/1 -> divide/2
  In1/1 -> multiplica/1
  multiplica1/1 -> Display2/1, Integrator/1
  In4/1 -> Sum/1
  Sum/1 -> multiplica1/2
  divide/1 -> multiplica1/1
  In2/1 -> multiplica/2
  multiplica/1 -> divide/1
  Integrator/1 -> Display1/1, Out1/1, Sum/2

== system modeloKevin/Subsystem3 ==
  note: Tg
  note: dtg/dt
  In1 : Inport
  In2 : Inport  Port=2
  In3 : Inport  Port=3
  Divide2 : Product  Inputs=/*
  Divide3 : Product  Inputs=**
  Integrator : Integrator
  Sum1 : Sum  Inputs=|+-
  Out1 : Outport
  wires:
  Sum1/1 -> Divide3/1
  Integrator/1 -> Sum1/2, Out1/1
  In1/1 -> Sum1/1
  Divide2/1 -> Divide3/2
  In3/1 -> Divide2/2
  In2/1 -> Divide2/1
  Divide3/1 -> Integrator/1

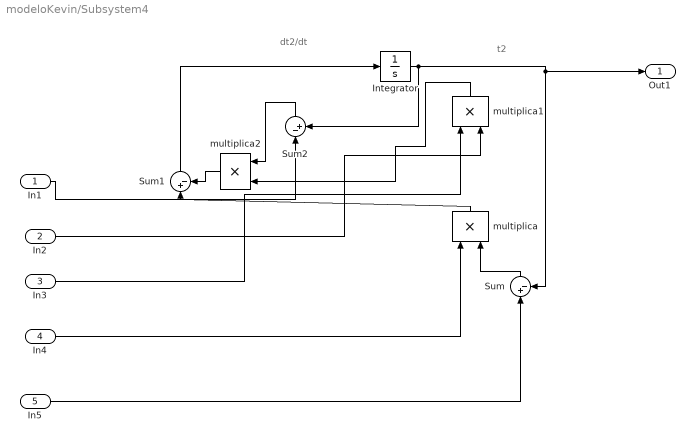
== system modeloKevin/Subsystem4 ==
  note: dt2/dt
  note: t2
  In1 : Inport
  In2 : Inport  Port=2
  In3 : Inport  Port=3
  In4 : Inport  Port=4
  In5 : Inport  Port=5
  Integrator : Integrator
  Sum : Sum  Inputs=|+-
  Sum1 : Sum  Inputs=|+-
  Sum2 : Sum  Inputs=|-+
  multiplica : Product  Inputs=**
  multiplica1 : Product  Inputs=**
  multiplica2 : Product  Inputs=**
  Out1 : Outport
  wires:
  Sum/1 -> multiplica/2
  In3/1 -> multiplica1/1
  multiplica2/1 -> Sum1/2
  In2/1 -> multiplica1/2
  multiplica1/1 -> multiplica2/2
  multiplica/1 -> Sum1/1
  Integrator/1 -> Sum2/2, Out1/1, Sum/2
  In4/1 -> multiplica/1
  Sum2/1 -> multiplica2/1
  In1/1 -> Sum2/1
  In5/1 -> Sum/1
  Sum1/1 -> Integrator/1

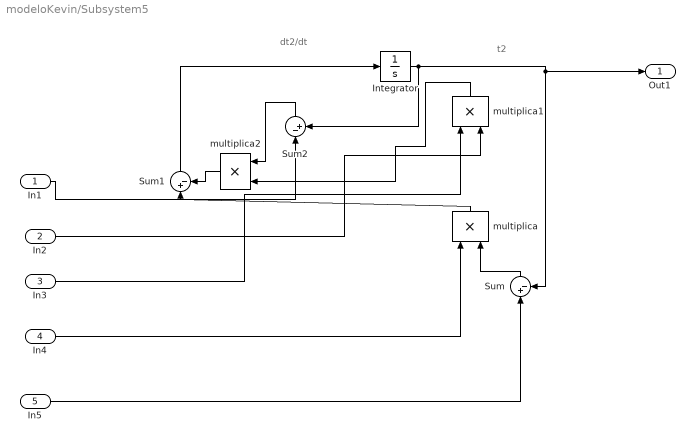
== system modeloKevin/Subsystem5 ==
  note: dt2/dt
  note: t2
  In1 : Inport
  In2 : Inport  Port=2
  In3 : Inport  Port=3
  In4 : Inport  Port=4
  In5 : Inport  Port=5
  Integrator : Integrator
  Sum : Sum  Inputs=|+-
  Sum1 : Sum  Inputs=|+-
  Sum2 : Sum  Inputs=|-+
  multiplica : Product  Inputs=**
  multiplica1 : Product  Inputs=**
  multiplica2 : Product  Inputs=**
  Out1 : Outport
  wires:
  Sum/1 -> multiplica/2
  In3/1 -> multiplica1/1
  multiplica2/1 -> Sum1/2
  In2/1 -> multiplica1/2
  multiplica1/1 -> multiplica2/2
  multiplica/1 -> Sum1/1
  Integrator/1 -> Sum2/2, Out1/1, Sum/2
  In4/1 -> multiplica/1
  Sum2/1 -> multiplica2/1
  In1/1 -> Sum2/1
  In5/1 -> Sum/1
  Sum1/1 -> Integrator/1

== system modeloKevin/Subsystem6 ==
  In1 : Inport
  In2 : Inport  Port=2
  Gain6 : Gain  Gain=2*pi
  Product8 : Product
  Out1 : Outport
  wires:
  Product8/1 -> Out1/1
  In2/1 -> Product8/2
  Gain6/1 -> Product8/1
  In1/1 -> Gain6/1

== system modeloKevin/Subsystem7 ==
  In1 : Inport
  In2 : Inport  Port=2
  In3 : Inport  Port=3
  In4 : Inport  Port=4
  Divide : Product  Inputs=**
  Sum3 : Sum  Inputs=|++
  Sum4 : Sum  Inputs=|++
  Out1 : Outport
  wires:
  In2/1 -> Sum3/2
  Sum3/1 -> Sum4/1
  In4/1 -> Divide/2
  In3/1 -> Sum4/2
  In1/1 -> Sum3/1
  Divide/1 -> Out1/1
  Sum4/1 -> Divide/1

== system modeloKevin/Subsystem8 ==
  In1 : Inport
  In2 : Inport  Port=2
  Gain8 : Gain  Gain=2*pi
  Product9 : Product
  Out1 : Outport
  wires:
  In2/1 -> Product9/2
  In1/1 -> Gain8/1
  Product9/1 -> Out1/1
  Gain8/1 -> Product9/1

== system modeloKevin/Subsystem9 ==
  In1 : Inport
  In2 : Inport  Port=2
  In3 : Inport  Port=3
  In4 : Inport  Port=4
  divide : Product  Inputs=**
  divide1 : Product  Inputs=**
  divide2 : Product  Inputs=*/
  Out1 : Outport
  wires:
  divide/1 -> divide1/1
  In3/1 -> divide1/2
  In1/1 -> divide/1
  In2/1 -> divide/2
  In4/1 -> divide2/2
  divide2/1 -> Out1/1
  divide1/1 -> divide2/1

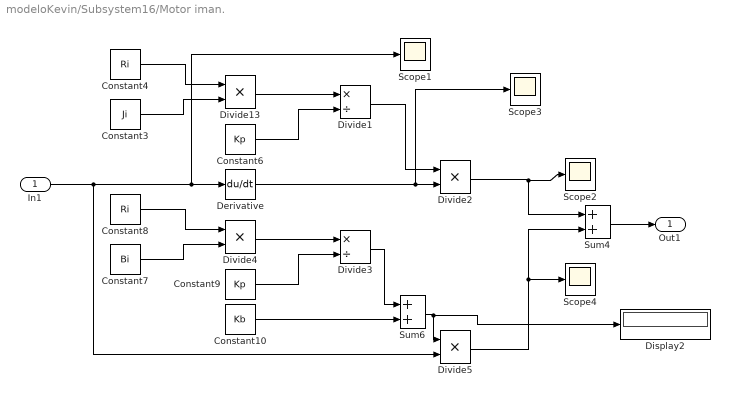
== system modeloKevin/Subsystem16/Motor iman. ==
  In1 : Inport
  Constant10 : Constant  Value=Kb
  Constant3 : Constant  Value=Ji
  Constant4 : Constant  Value=Ri
  Constant6 : Constant  Value=Kp
  Constant7 : Constant  Value=Bi
  Constant8 : Constant  Value=Ri
  Constant9 : Constant  Value=Kp
  Derivative : Derivative
  Display2 : Display
  Divide1 : Product  Inputs=*/  SaturateOnIntegerOverflow=on  RndMeth=Zero
  Divide{2,4..5,13} (4 alike) : Product  Inputs=**  SaturateOnIntegerOverflow=on  RndMeth=Zero
  Divide3 : Product  Inputs=*/  SaturateOnIntegerOverflow=on  RndMeth=Zero
  Scope{1..4} (4 alike) : Scope
  Sum4 : Sum
  Sum6 : Sum
  Out1 : Outport
  wires:
  Constant10/1 -> Sum6/2
  Divide2/1 -> Scope2/1, Sum4/1
  In1/1 -> Divide5/2, Scope1/1, Derivative/1
  Divide3/1 -> Sum6/1
  Divide13/1 -> Divide1/1
  Constant6/1 -> Divide1/2
  Constant4/1 -> Divide13/1
  Sum6/1 -> Display2/1, Divide5/1
  Divide1/1 -> Divide2/1
  Constant3/1 -> Divide13/2
  Constant9/1 -> Divide3/2
  Divide4/1 -> Divide3/1
  Constant7/1 -> Divide4/2
  Constant8/1 -> Divide4/1
  Derivative/1 -> Scope3/1, Divide2/2
  Sum4/1 -> Out1/1
  Divide5/1 -> Scope4/1, Sum4/2

== system modeloKevin/Subsystem16/Subsystem1 ==
  In1 : Inport
  Constant2 : Constant  Value=Kp
  Divide2 : Product  Inputs=**
  Out1 : Outport
  wires:
  In1/1 -> Divide2/1
  Constant2/1 -> Divide2/2
  Divide2/1 -> Out1/1

== system modeloKevin/Subsystem16/Subsystem2 ==
  In1 : Inport
  Constant : Constant  Value=CargaR
  Divide1 : Product  Inputs=*/
  Out1 : Outport
  wires:
  Divide1/1 -> Out1/1
  Constant/1 -> Divide1/2
  In1/1 -> Divide1/1

== matlab function modeloKevin/MATLAB Function1 ==
  data: T1 input; y1 output; T2 input; t input
function y1 = fcn(T1,T2,t)

% Initialize number of nodes and constants
N = 45;
ku = 15; % AISI 304 con ductividad termimica
rho = 7830; % AISI 304 densidad
cp = 500; % AISI 304 calor espe
L = 0.04;
q = 0;
h = L/(N-1); %delta de x
alfa=ku/(cp*rho);
dt = (0.5*(h^2))/alfa;
t = 20;
Ti = 300;
T0 = T2;
TL = T1;
r = (ku*dt)/(rho*cp*h^2);
if r>0.5
 error('disminuya el intervalo de tiempo dt')
end
% ubicaciÛn de los nodos
x = linspace(0,h,L);
% Temperatura incial en t = 0
jmax = round(t/dt);
u = zeros(N,jmax);
u(:,1) = Ti*ones(1,N);

u(1,:) = T0;
u(N,:) = TL;
for j = 1:jmax-1
 for i=2:N-1
 u(i,j+1) = (r*u(i-1,j)+(1-2*r)*u(i,j)+r*u(i+1,j)) + q*dt;
 end
end
%plot(u)
TW1=u(40,end);
y1=TW1;

== matlab function modeloKevin/MATLAB Function5 ==
  data: T11 input; Y output; T22 input; Tgw input; pcs input
function Y=fcn(T11,T22,Tgw,pcs)
u=0;
if pcs==1;
    u=Tgw;
end 

if pcs==2;
    u=T22;
end 

if pcs==3;
    u=Tgw;
end 

if pcs==4;
    u=T11;
end 

Y=u;

% pcs 1 calentamiento = Tgw
% pcs 2 expansion = Tge
% pcs 3 enfriamiento = Tgw
% pcs 4 compresion = Tgc

== matlab function modeloKevin/MATLAB Function2 ==
  data: T1 input; y2 output; T2 input; t input
function y2 = fcn(T1,T2,t)

% Initialize number of nodes and constants
N = 45;
ku = 15; % AISI 304 con ductividad termimica
rho = 7830; % AISI 304 densidad
cp = 500; % AISI 304 calor espe
L = 0.04;
q = 0;
h = L/(N-1); %delta de x
alfa=ku/(cp*rho);
dt = (0.5*(h^2))/alfa;
t = 20;
Ti = 300;
T0 = T2;
TL = T1;
r = (ku*dt)/(rho*cp*h^2);
if r>0.5
 error('disminuya el intervalo de tiempo dt')
end
% ubicaciÛn de los nodos
x = linspace(0,h,L);
% Temperatura incial en t = 0
jmax = round(t/dt);
u = zeros(N,jmax);
u(:,1) = Ti*ones(1,N);

u(1,:) = T0;
u(N,:) = TL;
for j = 1:jmax-1
 for i=2:N-1
 u(i,j+1) = (r*u(i-1,j)+(1-2*r)*u(i,j)+r*u(i+1,j)) + q*dt;
 end
end
%plot(u)
TW2=u(30,end);
y2=TW2;

== matlab function modeloKevin/MATLAB Function3 ==
  data: tetha input; y output
function y = fcn(tetha)


y=floor(4*((tetha/(2*3.1426))-floor(tetha/(2*3.1426))))+1;

== matlab function modeloKevin/MATLAB Function4 ==
  data: T1 input; y3 output; T2 input; t input
function y3 = fcn(T1,T2,t)

% Initialize number of nodes and constants
N = 45;
ku = 15; % AISI 304 con ductividad termimica
rho = 7830; % AISI 304 densidad
cp = 500; % AISI 304 calor espe
L = 0.04;
q = 0;
h = L/(N-1); %delta de x
alfa=ku/(cp*rho);
dt = (0.5*(h^2))/alfa;
t = 20;
Ti = 300;
T0 = T2;
TL = T1;
r = (ku*dt)/(rho*cp*h^2);
if r>0.5
 error('disminuya el intervalo de tiempo dt')
end
% ubicaciÛn de los nodos
x = linspace(0,h,L);
% Temperatura incial en t = 0
jmax = round(t/dt);
u = zeros(N,jmax);
u(:,1) = Ti*ones(1,N);

u(1,:) = T0;
u(N,:) = TL;
for j = 1:jmax-1
 for i=2:N-1
 u(i,j+1) = (r*u(i-1,j)+(1-2*r)*u(i,j)+r*u(i+1,j)) + q*dt;
 end
end
%plot(u)
TW3=u(20,end);

y3=TW3;

== matlab function modeloKevin/MATLAB Function6 ==
  data: T1 input; Twg output; T2 input; T3 input; T4 input; Xg input
function Twg = fcn(T1,T2,T3,T4,Xg)
u=0;
a=0.0337;
b=0.040;
c=0.0482;
d=0.0555;
e=0.0639;



if  (a<Xg) && (Xg<=b)
    
u=T1;
end

if (b<Xg) && (Xg<=c)
    
    u=T2;
end

if  (c<Xg) && (Xg<=d)
    
    u=T3;
end
if (d<Xg) && (Xg<=e)
    
    u=T4;
end

Twg=u;

== matlab function modeloKevin/MATLAB Function7 ==
  data: T1 input; y4 output; T2 input; t input
function y4 = fcn(T1,T2,t)

% Initialize number of nodes and constants
N = 45;
ku = 15; % AISI 304 con ductividad termimica
rho = 7830; % AISI 304 densidad
cp = 500; % AISI 304 calor espe
L = 0.04;
q = 0;
h = L/(N-1); %delta de x
alfa=ku/(cp*rho);
dt = (0.5*(h^2))/alfa;
t = 20;
Ti = 300;
T0 = T2;
TL = T1;
r = (ku*dt)/(rho*cp*h^2);
if r>0.5
 error('disminuya el intervalo de tiempo dt')
end
% ubicaciÛn de los nodos
x = linspace(0,h,L);
% Temperatura incial en t = 0
jmax = round(t/dt);
u = zeros(N,jmax);
u(:,1) = Ti*ones(1,N);

u(1,:) = T0;
u(N,:) = TL;
for j = 1:jmax-1
 for i=2:N-1
 u(i,j+1) = (r*u(i-1,j)+(1-2*r)*u(i,j)+r*u(i+1,j)) + q*dt;
 end
end
%plot(u)
TW4=u(1,end);

y4=TW4;
